simulink model "Serial"  (R2014a)
settings: Solver=FixedStepDiscrete  StartTime=0.0  StopTime=inf  FixedStep=0.06  RelTol=1e-3
libraries: simulink x6
settings Model: SimulationMode=external  ExtModeTrigDuration=100  Creator=jsustare  LastModifiedBy=jsustare
settings OptimizationCC: OptimizeModelRefInitCode=on  LifeSpan=1
settings DebuggingCC: UnderspecifiedInitializationDetection=Classic  SolverPrmCheckMsg=none
settings HardwareCC: ProdLargestAtomicInteger=Long  ProdLargestAtomicFloat=Double  ProdEndianess=LittleEndian  ProdHWDeviceType=ARM Compatible->ARM Cortex
settings RTWCC: SystemTargetFile=realtime.tlc  GenerateMakefile=off  TemplateMakefile=realtime.tmf  Description=Run on Target Hardware  RTWVerbose=off  ProcessScript=realtime_make_rtw_hook  CustomInclude=include include/common  CustomSource=SerialPort.c mavlink.c
settings RTWCC: CustomHeaderCode=|
  | #include <mavlink.h>
  | #include <common.h>
settings STFCustomTargetCC: TargetLibSuffix=.a  GenerateSampleERTMain=on  ConcurrentExecutionCompliant=off  GeneratePreprocessorConditionals=Use local settings  ERTCustomFileBanners=on  SupportNonInlinedSFcns=off  SupportVariableSizeSignals=on  MATLABClassNameForMDSCustomization=Simulink.SoftwareTarget.ERTCustomization  GRTInterface=off  SystemTargetFile=realtime.tlc
settings ERTTargetCC: CombineOutputUpdateFcns=off  SupportContinuousTime=on  SupportVariableSizeSignals=on  ExtModeMexArgs='169.254.0.31' 0 17725  ERTSrcFileBannerTemplate=realtime_code_template.cgt  ERTHdrFileBannerTemplate=realtime_code_template.cgt  ERTDataSrcFileTemplate=realtime_code_template.cgt  ERTDataHdrFileTemplate=realtime_code_template.cgt  ERTCustomFileTemplate=realtime_file_process.tlc

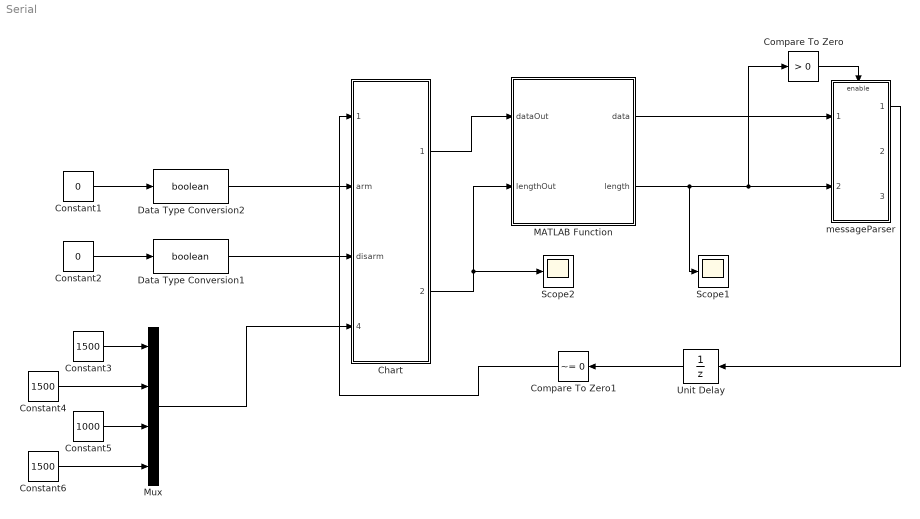
== system Serial ==
  Chart : Stateflow chart  TreatAsAtomicUnit=on
  Compare To Zero : simulink/Logic and Bit Operations/Compare To Zero  relop=>  OutDataTypeStr=boolean
  Compare To Zero1 : simulink/Logic and Bit Operations/Compare To Zero  relop=~=  OutDataTypeStr=boolean
  Constant1 : Constant  Value=0
  Constant2 : Constant  Value=0
  Constant3 : Constant  Value=1500
  Constant4 : Constant  Value=1500
  Constant5 : Constant  Value=1000
  Constant6 : Constant  Value=1500
  Data Type Conversion1 : DataTypeConversion  OutDataTypeStr=boolean
  Data Type Conversion2 : DataTypeConversion  OutDataTypeStr=boolean
  MATLAB Function : MATLAB Function  TreatAsAtomicUnit=on
  Mux : Mux
  Scope1 : Scope
      settings: YMin=0  YMax=50  SaveName=ScopeData2
  Scope2 : Scope
      settings: YMin=13.3  YMax=14.7
  Unit Delay : UnitDelay  SampleTime=-1
  messageParser : Subsystem
  wires:
  MATLAB Function/2(length) -> Scope1/1, Compare To Zero/1, messageParser/2(lengthRead)
  Compare To Zero/1 -> messageParser/Enable
  Chart/1(dataOut) -> MATLAB Function/1(dataOut)
  Chart/2(lengthOut) -> MATLAB Function/2(lengthOut), Scope2/1
  Unit Delay/1 -> Compare To Zero1/1
  Compare To Zero1/1 -> Chart/1(dataReceived)
  Constant1/1 -> Data Type Conversion2/1
  Data Type Conversion2/1 -> Chart/2(arm)
  Constant2/1 -> Data Type Conversion1/1
  Data Type Conversion1/1 -> Chart/3(disarm)
  Mux/1 -> Chart/4(PRYTvals)
  Constant3/1 -> Mux/1
  Constant4/1 -> Mux/2
  Constant5/1 -> Mux/3
  Constant6/1 -> Mux/4
  MATLAB Function/1(data) -> messageParser/1("dataRead ")
  messageParser/1(dataBeingReceived) -> Unit Delay/1

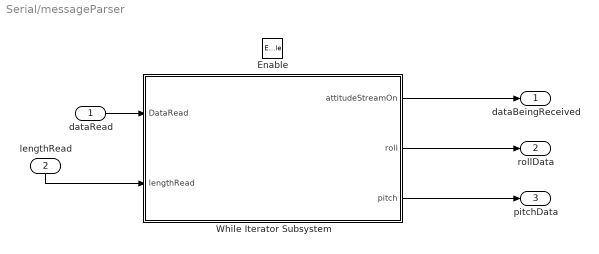
== system Serial/messageParser ==
  "dataRead " : Inport
  lengthRead : Inport  Port=2
  Enable : EnablePort
  While Iterator Subsystem : Subsystem  TreatAsAtomicUnit=on
  dataBeingReceived : Outport
  rollData : Outport  Port=2
  pitchData : Outport  Port=3
  wires:
  "dataRead "/1 -> While Iterator Subsystem/1(DataRead)
  While Iterator Subsystem/1(attitudeStreamOn) -> dataBeingReceived/1
  lengthRead/1 -> While Iterator Subsystem/2(lengthRead)
  While Iterator Subsystem/2(roll) -> rollData/1
  While Iterator Subsystem/3(pitch) -> pitchData/1

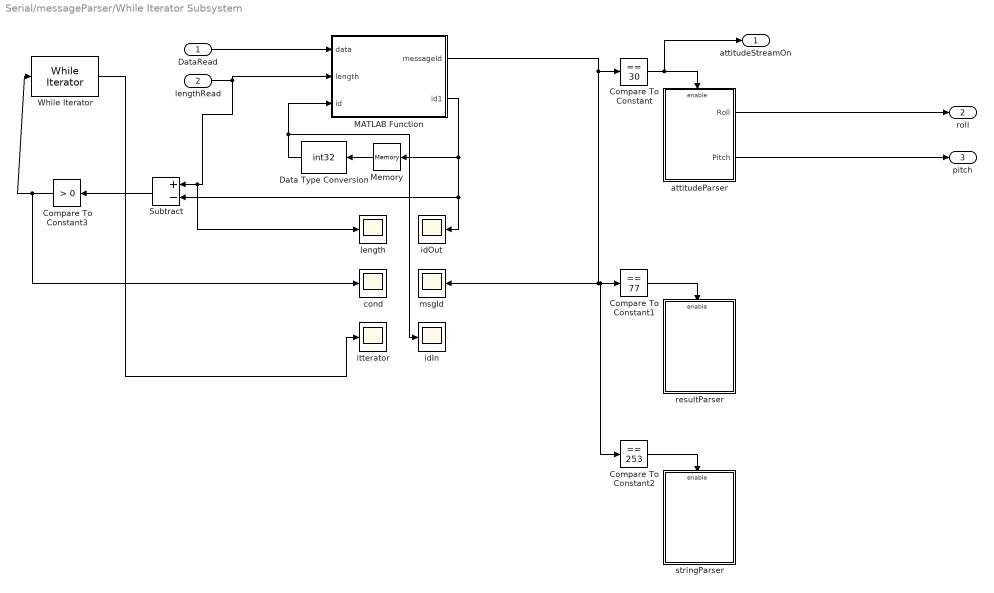
== system Serial/messageParser/While Iterator Subsystem ==
  DataRead : Inport
  lengthRead : Inport  Port=2
  Compare To Constant : simulink/Logic and Bit Operations/Compare To Constant  relop===  const=30  OutDataTypeStr=boolean
  Compare To Constant1 : simulink/Logic and Bit Operations/Compare To Constant  relop===  const=77  OutDataTypeStr=boolean
  Compare To Constant2 : simulink/Logic and Bit Operations/Compare To Constant  relop===  const=253  OutDataTypeStr=boolean
  Compare To Constant3 : simulink/Logic and Bit Operations/Compare To Constant  relop=>  const=0  OutDataTypeStr=boolean
  Data Type Conversion : DataTypeConversion  OutDataTypeStr=int32
  MATLAB Function : MATLAB Function  TreatAsAtomicUnit=on
  Memory : Memory  X0=1  InheritSampleTime=on
  Subtract : Sum  Inputs=+-
  While Iterator : WhileIterator  MaxIters=100  WhileBlockType=do-while  ShowIterationPort=on
  attitudeParser : Subsystem
  cond : Scope
      settings: YMin=0.95  YMax=1.05  SaveName=ScopeData6
  idIn : Scope
      settings: TimeRange=10  YMin=0  YMax=40  SaveName=ScopeData8
  idOut : Scope
      settings: YMin=2.5  YMax=55  SaveName=ScopeData5
  "itterator " : Scope
      settings: TimeRange=10  YMin=1  YMax=1  SaveName=ScopeData3
  length : Scope
      settings: TimeRange=10  YMin=35  YMax=72.5  SaveName=ScopeData7
  msgId : Scope
  resultParser : Subsystem
  stringParser : Subsystem
  attitudeStreamOn : Outport
  roll : Outport  Port=2
  pitch : Outport  Port=3
  wires:
  Compare To Constant/1 -> attitudeStreamOn/1, attitudeParser/Enable
  Compare To Constant1/1 -> resultParser/Enable
  Compare To Constant2/1 -> stringParser/Enable
  MATLAB Function/1(messageId) -> Compare To Constant2/1, Compare To Constant1/1, msgId/1, Compare To Constant/1
  DataRead/1 -> MATLAB Function/1(data)
  lengthRead/1 -> length/1, Subtract/1, MATLAB Function/2(length)
  Compare To Constant3/1 -> cond/1, While Iterator/1
  attitudeParser/1("Roll\t") -> roll/1
  attitudeParser/2(Pitch) -> pitch/1
  While Iterator/1 -> "itterator "/1
  Memory/1 -> Data Type Conversion/1
  Data Type Conversion/1 -> MATLAB Function/3(id), idIn/1
  MATLAB Function/2(id1) -> Subtract/2, idOut/1, Memory/1
  Subtract/1 -> Compare To Constant3/1

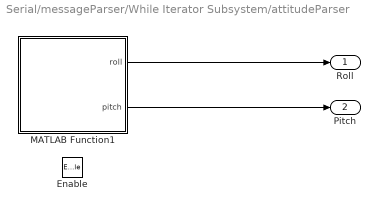
== system Serial/messageParser/While Iterator Subsystem/attitudeParser ==
  Enable : EnablePort
  MATLAB Function1 : MATLAB Function  TreatAsAtomicUnit=on
  "Roll\t" : Outport
  Pitch : Outport  Port=2
  wires:
  MATLAB Function1/2(pitch) -> Pitch/1
  MATLAB Function1/1(roll) -> "Roll\t"/1

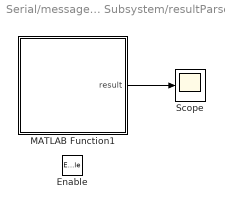
== system Serial/messageParser/While Iterator Subsystem/resultParser ==
  Enable : EnablePort
  MATLAB Function1 : MATLAB Function  TreatAsAtomicUnit=on
  Scope : Scope
      settings: SaveName=ScopeData4
  wires:
  MATLAB Function1/1(result) -> Scope/1

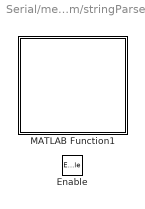
== system Serial/messageParser/While Iterator Subsystem/stringParser ==
  Enable : EnablePort
  MATLAB Function1 : MATLAB Function  TreatAsAtomicUnit=on

== matlab function Serial/messageParser/While Iterator Subsystem/MATLAB Function ==
  data: data input; messageId output; length input; id input; id1 output
function [messageId,id1]  = parseMavlink(data, length, id)
messageId=uint8(0);
id1=int32(1);
if ~coder.target('SFun')
    for i=id:length
        tempD=uint8(0);
        tempD=coder.ceval('parseMavlink',data(i));         
        if tempD>0
            messageId = coder.ceval('getMessageId',i,length);
            if i==length
                id1=i;
            else
                id1=i+1;
            end            
            break;
        else
            id1=i;% if itteration finishes without id trigger - 
        end         
    end     
end
%% remarks ask Owen
% after implementing this  and when it was finally working the latency was 
% crazy(it was reading attitude at irregular frequency  with up to 2 sec lag). but 
% when model execution step size was increased(from 0.02 to 0.05) ie executed slower 
% then latency decreased. why? is it because whe while loop executes slowly ? 
% and that was causing the whole model to lag? or maybe it wasnt getting full messages?
% but attitude data was suppose to be 50Hz.  
%% new issue probably explains the above 
% this now read the data from serial, looks from message id and parses all 
% the messages whos id it finds. if the data from serial ends midway a message,
% then id is not found and this first part of the message is discarded after
% end of data is reached

== matlab function Serial/MATLAB Function ==
  data: data output; length output; dataOut input; lengthOut input
function [data, length] = serialReadWrite(dataOut, lengthOut)
persistent spHandle;
data = zeros(512,1,'uint8');
length =int32(0);
if ~coder.target('SFun')
    if isempty(spHandle)
        spHandle = int32(0);
        spHandle =coder.ceval('setupSerialPort',['/dev/ttyAMA0' 0], uint32(57600));
    end
    if spHandle>0
        bytesRead = int32(0);
        dataRead = zeros(512,1,'uint8');
        bytesRead = coder.ceval('read',spHandle, coder.ref(dataRead), uint32(256));
        if bytesRead>0
            data= dataRead;
            length=bytesRead;
        end
        if lengthOut>0
            bytesWritten = int32(0);
            data2=uint8(dataOut);
            bytesWritten= coder.ceval('write',spHandle, coder.ref(data2), uint32(lengthOut));
        end
    end
end

== matlab function Serial/messageParser/While Iterator Subsystem/resultParser/MATLAB Function1 ==
  data: result output
function result  = parseResult
result=uint8(0);
if ~coder.target('SFun')
    coder.ceval('getResult',coder.ref(result));    
end

== matlab function Serial/messageParser/While Iterator Subsystem/attitudeParser/MATLAB Function1 ==
  data: roll output; pitch output
function [roll,pitch] = parseRollPitch()
roll=double(0);
pitch=double(0);
if ~coder.target('SFun')
    coder.ceval('getRoll',coder.ref(roll));
    coder.ceval('getPitch',coder.ref(pitch));
end

== stateflow chart Serial/Chart ==
  state Initializing
    entry:[dataOut,lengthOut] = requestStreams;
    exit:lengthOut=uint8(0);
  state Disarmed
    state sendDisarm
      entry:[dataOut,lengthOut] = sendArmDisarmFun(0);
      exit:lengthOut=uint8(0);
    state idle
    (default) -> sendDisarm
    sendDisarm -> idle : after(1,sec')
  state Armed
    state sendArm
      entry:[dataOut,lengthOut] = sendArmDisarmFun(1);
      exit:lengthOut=uint8(0);
    state Flying
      during:[dataOut,lengthOut] =sendRPYT(PRYTvals(1),...
      PRYTvals(2),PRYTvals(3),PRYTvals(4));
    (default) -> sendArm
    sendArm -> Flying : after(1,sec)
  (default) -> Initializing
  Initializing -> Disarmed : [dataReceived]
  Armed -> Disarmed : [disarm]
  Disarmed -> Armed : [arm]
  data: data function_output; length function_output; data function_output; length function_output; armdisarm function_input; data function_output; length function_output; R function_input; P function_input; Y function_input; T function_input; dataOut output; lengthOut output; dataReceived input; arm input; disarm input; PRYTvals input size=4
  function [data,length] = requestStreams:
    | function  [data,length] = requestStreams
    | data2 = zeros(256,1,'uint8');
    | length =uint8(0);
    | data=data2;
    | if ~coder.target('SFun')
    |   length=coder.ceval('requestAttitude', coder.ref(data2));
    |   data=data2;
    | end
  function [data,length] = sendArmDisarmFun(armdisarm):
    | function  [data,length] = sendArmDisarmFun(armdisarm)
    | data2 = zeros(256,1,'uint8');
    | length =uint8(0);
    | data=data2;
    | if ~coder.target('SFun')
    |   length=coder.ceval('sendArmDisarm', coder.ref(data2),uint8(armdisarm));
    |   data=data2;
    | end
  function [data,length] = sendRPYT(R, P, Y, T):
    | function  [data,length] = sendRPYT(R, P, Y, T)
    | data2 = zeros(256,1,'uint8');
    | length =uint8(0);
    | data=data2;
    | if ~coder.target('SFun')
    |     length=coder.ceval('sendRPYT',...
    |         coder.ref(data2),uint16(R),uint16(P),uint16(Y),uint16(T));
    |     data=data2;
    | end

== matlab function Serial/messageParser/While Iterator Subsystem/stringParser/MATLAB Function1 ==
function parseString
if ~coder.target('SFun')
    coder.ceval('getString');    
end
